simulink model "sampleModel1798"  (R2023a)
settings: Solver=VariableStepAuto  StartTime=0.0  StopTime=10.0  RelTol=1e-3
libraries: hdlsllib x6, simulink x2
settings Model: Creator=user1  LastModifiedBy=user1

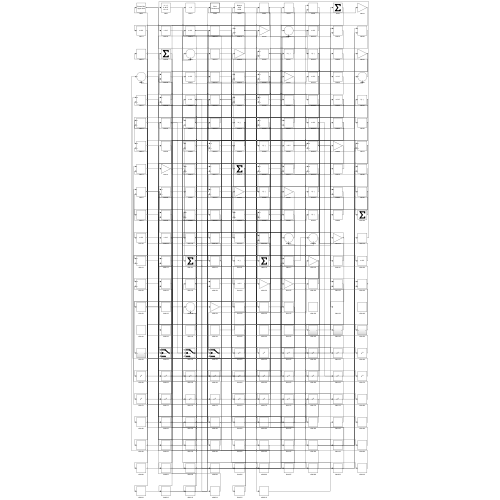
[thumbnail: Simulink's stored preview of the top-level diagram]
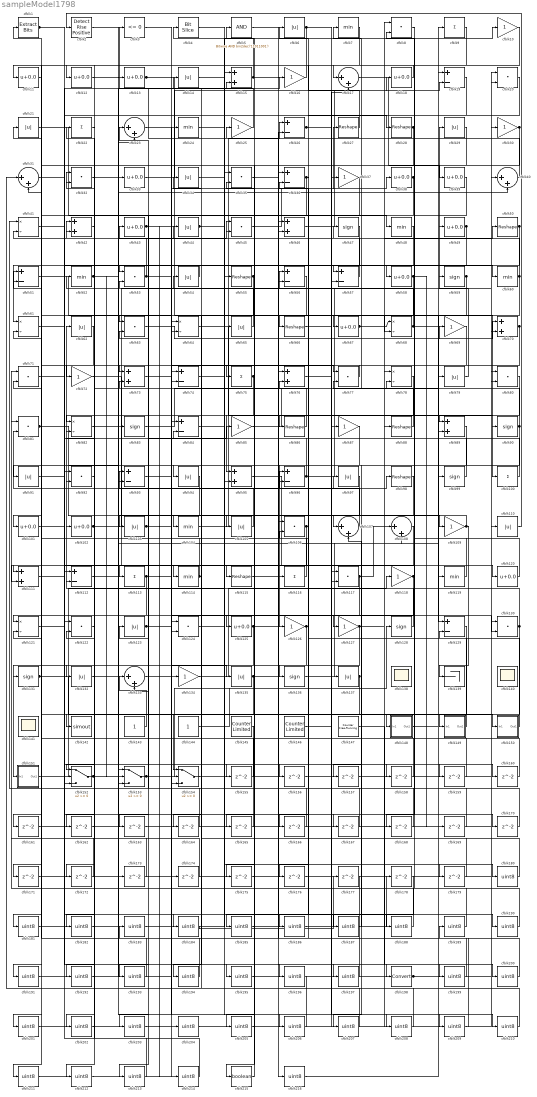
== system sampleModel1798 ==
  cfblk1 : simulink/Logic and Bit Operations/Extract Bits  bitsToExtract=Upper half  numBits=8  bitIdxRange=[0 7]  outScalingMode=Preserve fixed-point scaling
      settings: LibrarySourceBlock=|
      | hdlsllib/Logic and Bit
      | Operations/Extract Bits
  cfblk{10,16,25,30,37,69,72,85,87,109,118,126..127,134} (14 alike) : Gain
  cfblk{9,22,75,100,113,116} (6 alike) : Sum  Inputs=+
  cfblk{11..13,18,33,38..39,43,49,58,67,101..102,120,125} (15 alike) : Bias  Bias=0.0  SaturateOnIntegerOverflow=off
  cfblk{6,14,21,29,34,44,54,62,65,79,91,94,97,103,105,110,123,132,135,137} (20 alike) : Abs  SaturateOnIntegerOverflow=off
  cfblk{7,24,48,52,60,104,114,119} (8 alike) : MinMax
  cfblk{8,20,32,35,45,53,63,71,77,80..81,92,106,117,122,124,130} (17 alike) : DotProduct  OutDataTypeStr=Inherit: Inherit via internal rule
  cfblk{17,23,31,40,107..108,133} (7 alike) : Sum  Inputs=|++
  cfblk{15,42,46,70,73,76,89,95,111} (9 alike) : Sum
  cfblk{19,26,36,51,56..57,74,84,93,96,112,129} (12 alike) : Sum  Inputs=+-
  cfblk{27..28,50,55,66,86,88,98,115} (9 alike) : Reshape
  cfblk{41,61,64,68,78,82,121} (7 alike) : Product  Inputs=*/  RndMeth=Zero  SaturateOnIntegerOverflow=on
  cfblk{47,59,83,90,99,128,131,136} (8 alike) : Signum
  cfblk138 : Scope
      settings: Floating=on
  cfblk139 : Terminator
  cfblk140 : Scope
      settings: Floating=on
  cfblk141 : Scope
      settings: Floating=on
  cfblk142 : ToWorkspace  VariableName=simout  SaveFormat=Timeseries  SampleTime=-1
  cfblk143 : Constant  SampleTime=-1
  cfblk144 : Constant  SampleTime=-1
  cfblk145 : hdlsllib/Sources/Counter Limited  uplimit=7  tsamp=-1
  cfblk146 : hdlsllib/Sources/Counter Limited  uplimit=7  tsamp=-1
  cfblk147 : hdlsllib/Sources/Counter Free-Running  NumBits=16  tsamp=-1
  cfblk148 : Subsystem
      settings: LibrarySourceBlock=|
      | hdlsllib/Ports &
      | Subsystems/Subsystem
  cfblk149 : Subsystem
      settings: LibrarySourceBlock=|
      | hdlsllib/Ports &
      | Subsystems/Subsystem
  cfblk150 : Subsystem
      settings: LibrarySourceBlock=|
      | hdlsllib/Ports &
      | Subsystems/Subsystem
  cfblk151 : Subsystem
      settings: LibrarySourceBlock=|
      | hdlsllib/Ports &
      | Subsystems/Subsystem
  cfblk152 : Switch  SaturateOnIntegerOverflow=off  InputSameDT=off
  cfblk153 : Switch  SaturateOnIntegerOverflow=off  InputSameDT=off
  cfblk154 : Switch  SaturateOnIntegerOverflow=off  InputSameDT=off
  cfblk{155..179} (25 alike) : Delay  SampleTime=1
  cfblk{180..197,199..214,216} (35 alike) : DataTypeConversion  OutDataTypeStr=uint8  SaturateOnIntegerOverflow=off  RndMeth=Floor
  cfblk198 : DataTypeConversion  SaturateOnIntegerOverflow=off  RndMeth=Floor
  cfblk2 : hdlsllib/Logic and Bit Operations/Detect Rise Positive  vinit=0  OutDataTypeStr=boolean
  cfblk215 : DataTypeConversion  OutDataTypeStr=boolean  SaturateOnIntegerOverflow=off  RndMeth=Floor
  cfblk3 : hdlsllib/Logic and Bit Operations/Compare To Zero  relop=<=  OutDataTypeStr=boolean
  cfblk4 : hdlsllib/Logic and Bit Operations/Bit Slice  lidx=7  ridx=0
  cfblk5 : simulink/Logic and Bit Operations/Bitwise Operator  logicop=AND  UseBitMask=on  BitMask=bin2dec('11011001')  BitMaskRealWorld=Stored Integer
      settings: LibrarySourceBlock=|
      | hdlsllib/Logic and Bit
      | Operations/Bitwise
      | Operator
  wires:
  cfblk21/1 -> cfblk48/1
  cfblk8/1 -> cfblk113/1
  cfblk54/1 -> cfblk53/1
  cfblk46/1 -> cfblk19/2
  cfblk153/1 -> cfblk128/1, cfblk123/1, cfblk210/1
  cfblk76/1 -> cfblk198/1
  cfblk127/1 -> cfblk49/1, cfblk171/1
  cfblk72/1 -> cfblk126/1
  cfblk25/1 -> cfblk3/1
  cfblk85/1 -> cfblk9/1
  cfblk47/1 -> cfblk61/1
  cfblk102/1 -> cfblk29/1, cfblk108/2
  cfblk128/1 -> cfblk62/1
  cfblk145/1 -> cfblk41/1
  cfblk98/1 -> cfblk104/1
  cfblk131/1 -> cfblk149/1(In1), cfblk84/2
  cfblk108/1 -> cfblk115/1
  cfblk16/1 -> cfblk12/1
  cfblk17/1 -> cfblk39/1
  cfblk104/1 -> cfblk26/1
  cfblk64/1 -> cfblk89/1
  cfblk53/1 -> cfblk42/1, cfblk60/1
  cfblk15/1 -> cfblk4/1, cfblk68/2, cfblk150/1(In1)
  cfblk43/1 -> cfblk100/1, cfblk214/1
  cfblk50/1 -> cfblk41/2, cfblk93/2
  cfblk40/1 -> cfblk13/1
  cfblk52/1 -> cfblk16/1, cfblk153/2
  cfblk63/1 -> cfblk69/1
  cfblk118/1 -> cfblk131/1, cfblk207/1
  cfblk103/1 -> cfblk109/1, cfblk174/1
  cfblk107/1 -> cfblk42/2
  cfblk13/1 -> cfblk119/1, cfblk77/1
  cfblk137/1 -> cfblk205/1, cfblk211/1
  cfblk152/1 -> cfblk102/1, cfblk98/1
  cfblk77/1 -> cfblk72/1
  cfblk41/1 -> cfblk57/1
  cfblk110/1 -> cfblk2/1
  cfblk143/1 -> cfblk133/1
  cfblk57/1 -> cfblk45/1
  cfblk151/1(Out1) -> cfblk55/1
  cfblk51/1 -> cfblk134/1
  cfblk33/1 -> cfblk18/1
  cfblk9/1 -> cfblk57/2
  cfblk75/1 -> cfblk82/1, cfblk95/1
  cfblk73/1 -> cfblk38/1
  cfblk69/1 -> cfblk73/1
  cfblk60/1 -> cfblk132/1, cfblk21/1, cfblk163/1
  cfblk38/1 -> cfblk75/1, cfblk95/2
  cfblk30/1 -> cfblk136/1, cfblk125/1
  cfblk90/1 -> cfblk154/3, cfblk77/2, cfblk157/1
  cfblk99/1 -> cfblk54/1
  cfblk6/1 -> cfblk160/1, cfblk161/1, cfblk162/1
  cfblk106/1 -> cfblk36/2, cfblk111/2
  cfblk26/1 -> cfblk130/2, cfblk208/1
  cfblk3/1 -> cfblk107/1
  cfblk56/1 -> cfblk63/1
  cfblk20/1 -> cfblk58/1
  cfblk36/1 -> cfblk133/2, cfblk86/1
  cfblk82/1 -> cfblk83/1
  cfblk125/1 -> cfblk151/1(In1), cfblk167/1
  cfblk117/1 -> cfblk108/1, cfblk172/1
  cfblk83/1 -> cfblk78/2
  cfblk148/1(Out1) -> cfblk70/1
  cfblk88/1 -> cfblk7/1
  cfblk89/1 -> cfblk116/1
  cfblk130/1 -> cfblk93/1, cfblk176/1
  cfblk121/1 -> cfblk15/2
  cfblk100/1 -> cfblk34/1
  cfblk61/1 -> cfblk120/1
  cfblk45/1 -> cfblk27/1
  cfblk68/1 -> cfblk89/2, cfblk90/1, cfblk25/1
  cfblk126/1 -> cfblk96/1, cfblk154/2
  cfblk10/1 -> cfblk11/1
  cfblk49/1 -> cfblk103/1, cfblk175/1
  cfblk28/1 -> cfblk148/1(In1), cfblk182/1
  cfblk44/1 -> cfblk65/1, cfblk10/1
  cfblk150/1(Out1) -> cfblk56/1
  cfblk27/1 -> cfblk6/1
  cfblk116/1 -> cfblk23/1
  cfblk95/1 -> cfblk129/1
  cfblk120/1 -> cfblk52/1
  cfblk132/1 -> cfblk45/2
  cfblk149/1(Out1) -> cfblk129/2
  cfblk134/1 -> cfblk46/1
  cfblk65/1 -> cfblk43/1
  cfblk109/1 -> cfblk139/1, cfblk105/1
  cfblk136/1 -> cfblk99/1
  cfblk22/1 -> cfblk142/1
  cfblk18/1 -> cfblk17/1
  cfblk79/1 -> cfblk59/1
  cfblk105/1 -> cfblk81/2
  cfblk81/1 -> cfblk117/1, cfblk173/1
  cfblk58/1 -> cfblk94/1, cfblk168/1, cfblk169/1
  cfblk96/1 -> cfblk30/1, cfblk53/2
  cfblk144/1 -> cfblk117/2
  cfblk67/1 -> cfblk68/1, cfblk50/1
  cfblk114/1 -> cfblk51/1, cfblk194/1
  cfblk19/1 -> cfblk106/1
  cfblk23/1 -> cfblk84/1
  cfblk86/1 -> cfblk32/1
  cfblk119/1 -> cfblk47/1
  cfblk29/1 -> cfblk101/1
  cfblk4/1 -> cfblk67/1
  cfblk70/1 -> cfblk114/1, cfblk152/3
  cfblk11/1 -> cfblk91/1
  cfblk62/1 -> cfblk121/1
  cfblk1/1 -> cfblk28/1, cfblk188/1
  cfblk154/1 -> cfblk56/2
  cfblk48/1 -> cfblk64/2
  cfblk55/1 -> cfblk164/1, cfblk165/1, cfblk202/1
  cfblk42/1 -> cfblk22/1
  cfblk146/1 -> cfblk37/1
  cfblk135/1 -> cfblk118/1, cfblk154/1
  cfblk12/1 -> cfblk23/2
  cfblk113/1 -> cfblk97/1, cfblk85/1, cfblk153/3, cfblk204/1
  cfblk59/1 -> cfblk152/1, cfblk111/1
  cfblk32/1 -> cfblk40/2
  cfblk39/1 -> cfblk96/2
  cfblk14/1 -> cfblk66/1
  cfblk123/1 -> cfblk135/1, cfblk213/1
  cfblk93/1 -> cfblk127/1
  cfblk133/1 -> cfblk155/1
  cfblk155/1 -> cfblk1/1
  cfblk84/1 -> cfblk156/1
  cfblk156/1 -> cfblk19/1
  cfblk157/1 -> cfblk40/1
  cfblk101/1 -> cfblk158/1
  cfblk158/1 -> cfblk15/1
  cfblk115/1 -> cfblk159/1
  cfblk159/1 -> cfblk78/1
  cfblk160/1 -> cfblk36/1
  cfblk161/1 -> cfblk70/2
  cfblk162/1 -> cfblk46/2
  cfblk163/1 -> cfblk17/2
  cfblk164/1 -> cfblk63/2
  cfblk165/1 -> cfblk32/2
  cfblk7/1 -> cfblk166/1
  cfblk166/1 -> cfblk61/2
  cfblk167/1 -> cfblk51/2
  cfblk168/1 -> cfblk121/2
  cfblk169/1 -> cfblk73/2
  cfblk91/1 -> cfblk170/1
  cfblk170/1 -> cfblk153/1
  cfblk171/1 -> cfblk130/1
  cfblk172/1 -> cfblk81/1
  cfblk173/1 -> cfblk82/2
  cfblk174/1 -> cfblk152/2
  cfblk175/1 -> cfblk26/2
  cfblk176/1 -> cfblk106/2
  cfblk66/1 -> cfblk179/1
  cfblk179/1 -> cfblk14/1
  cfblk74/1 -> cfblk180/1
  cfblk180/1 -> cfblk35/2
  cfblk129/1 -> cfblk181/1
  cfblk181/1 -> cfblk74/1
  cfblk182/1 -> cfblk74/2
  cfblk177/1 -> cfblk183/1
  cfblk183/1 -> cfblk35/1
  cfblk2/1 -> cfblk184/1
  cfblk184/1 -> cfblk177/1
  cfblk178/1 -> cfblk185/1
  cfblk185/1 -> cfblk8/1
  cfblk97/1 -> cfblk186/1
  cfblk186/1 -> cfblk178/1
  cfblk71/1 -> cfblk187/1
  cfblk187/1 -> cfblk107/2
  cfblk188/1 -> cfblk71/1
  cfblk189/1 -> cfblk71/2
  cfblk24/1 -> cfblk190/1
  cfblk190/1 -> cfblk8/2
  cfblk37/1 -> cfblk191/1
  cfblk191/1 -> cfblk24/1
  cfblk122/1 -> cfblk192/1
  cfblk192/1 -> cfblk33/1
  cfblk94/1 -> cfblk193/1
  cfblk193/1 -> cfblk122/1
  cfblk194/1 -> cfblk122/2
  cfblk31/1 -> cfblk195/1
  cfblk195/1 -> cfblk20/2
  cfblk34/1 -> cfblk196/1
  cfblk196/1 -> cfblk31/1
  cfblk111/1 -> cfblk197/1
  cfblk197/1 -> cfblk31/2
  cfblk198/1 -> cfblk110/1, cfblk20/1
  cfblk147/1 -> cfblk199/1
  cfblk199/1 -> cfblk76/1
  cfblk35/1 -> cfblk200/1
  cfblk200/1 -> cfblk76/2
  cfblk87/1 -> cfblk201/1
  cfblk201/1 -> cfblk137/1
  cfblk202/1 -> cfblk87/1
  cfblk80/1 -> cfblk203/1
  cfblk203/1 -> cfblk88/1
  cfblk204/1 -> cfblk80/1
  cfblk205/1 -> cfblk80/2
  cfblk112/1 -> cfblk206/1
  cfblk206/1 -> cfblk44/1
  cfblk207/1 -> cfblk112/1
  cfblk208/1 -> cfblk112/2
  cfblk124/1 -> cfblk209/1
  cfblk209/1 -> cfblk189/1
  cfblk210/1 -> cfblk124/1
  cfblk211/1 -> cfblk124/2
  cfblk92/1 -> cfblk212/1
  cfblk212/1 -> cfblk64/1
  cfblk213/1 -> cfblk92/1
  cfblk214/1 -> cfblk92/2
  cfblk78/1 -> cfblk215/1
  cfblk215/1 -> cfblk5/1
  cfblk5/1 -> cfblk216/1
  cfblk216/1 -> cfblk79/1

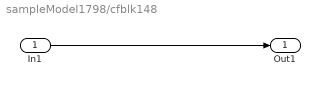
== system sampleModel1798/cfblk148 ==
  In1 : Inport
  Out1 : Outport
  wires:
  In1/1 -> Out1/1

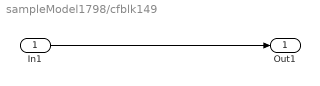
== system sampleModel1798/cfblk149 ==
  In1 : Inport
  Out1 : Outport
  wires:
  In1/1 -> Out1/1

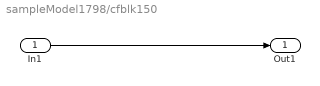
== system sampleModel1798/cfblk150 ==
  In1 : Inport
  Out1 : Outport
  wires:
  In1/1 -> Out1/1

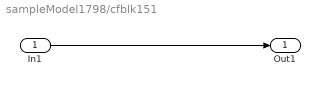
== system sampleModel1798/cfblk151 ==
  In1 : Inport
  Out1 : Outport
  wires:
  In1/1 -> Out1/1
